simulink model "control_strategy_2"  (R2024b)
settings: Solver=VariableStepAuto  StartTime=0.0  StopTime=5  MaxStep=1e-3  MinStep=1e-9  RelTol=1e-3
values from neighbouring files (symbols this model uses):
  C_filtre = 1 / (Lc * (2 * pi * 2000)^2)    (= 2.53302959106e-06)    [acdc_converter_parameters.m]
  Ccb = 330e-6    (= 0.00033)    [dcdc_converter_parameters.m]
  Cdc = 2200e-6    (= 0.0022)    [acdc_converter_parameters.m]
  Ci = 220e-6    (= 0.00022)    [dcdc_converter_parameters.m]
  Is = P / Vac    [acdc_converter_parameters.m]
  KI_curr_d = 2 * pi * w_i * rac    [acdc_converter_main.m]
  KI_curr_q = 2 * pi * w_i * rac    [acdc_converter_main.m]
  KI_out = KP_out * Wci_out    [dcdc_converter_main.m]
  KI_volt = C_volt.Ki    [acdc_converter_main.m]
  KIi = KPi * Wci_out    [dcdc_converter_main.m]
  KP_curr_d = 2 * pi * w_i * Lc    [acdc_converter_main.m]
  KP_curr_q = 2 * pi * w_i * Lc    [acdc_converter_main.m]
  KP_out = Wbi_volt / (Giod * Wci_out)    [dcdc_converter_main.m]
  KP_q = C_q.Kp    [acdc_converter_main.m]
  KP_volt = C_volt.Kp    [acdc_converter_main.m]
  KPi = Wbi_dc / (DCGain_iod * Wci_out)    [dcdc_converter_main.m]
  Lb = 3e-3    (= 0.003)    [dcdc_converter_parameters.m]
  Lc = 2.5e-3    (= 0.0025)    [acdc_converter_parameters.m]
  Lsi = 105e-6    (= 0.000105)    [dcdc_converter_parameters.m]
  P = 500    [main_control_strategy_2.m]
  phase = 0    [acdc_converter_parameters.m]
  Q = 0    [main_control_strategy_2.m]
  rac = 1e-3    (= 0.001)    [acdc_converter_parameters.m]
  rb = 1e-3    (= 0.001)    [dcdc_converter_parameters.m]
  ro = 270e-3    (= 0.27)    [dcdc_converter_parameters.m]
  Vb = 48    [dcdc_converter_parameters.m]
  Vdc = 200    [acdc_converter_parameters.m]
  Vdc0 = Vdc    (= 200)    [acdc_converter_parameters.m]
  Vs0 = Vac    (= 120)    [acdc_converter_parameters.m]
  w = 2 * pi * f    (= 376.991118431)    [acdc_converter_parameters.m]
  Zl = w * Lc    (= 0.942477796077)    [acdc_converter_parameters.m]
undefined symbols (not defined in the file or in its folder): q_switch, ri
libraries: spsSeriesRLCBranchLib x8, slpidlib x6, spsMosfetLib x6, spsVoltageMeasurementLib x5, spsMeanLib x4, spsParallelRLCBranchLib x3, spsCurrentMeasurementLib x3, spsTHDLib x3, spsDCVoltageSourceLib x2, spsACVoltageSourceLib x1, spsGroundLib x1, spsPWMGenerator2LevelLib x1
settings Model: Creator=casti  LastModifiedBy=Asus
settings OptimizationCC: ReuseModelBlockBuffer=off
settings RTWCC: GPUComputeCapability=3.5

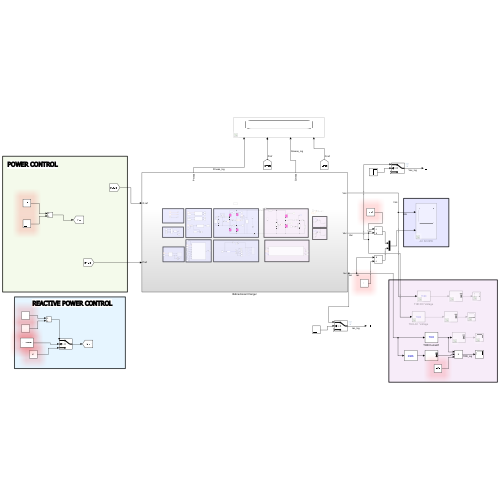
[thumbnail: Simulink's stored preview of the top-level diagram]
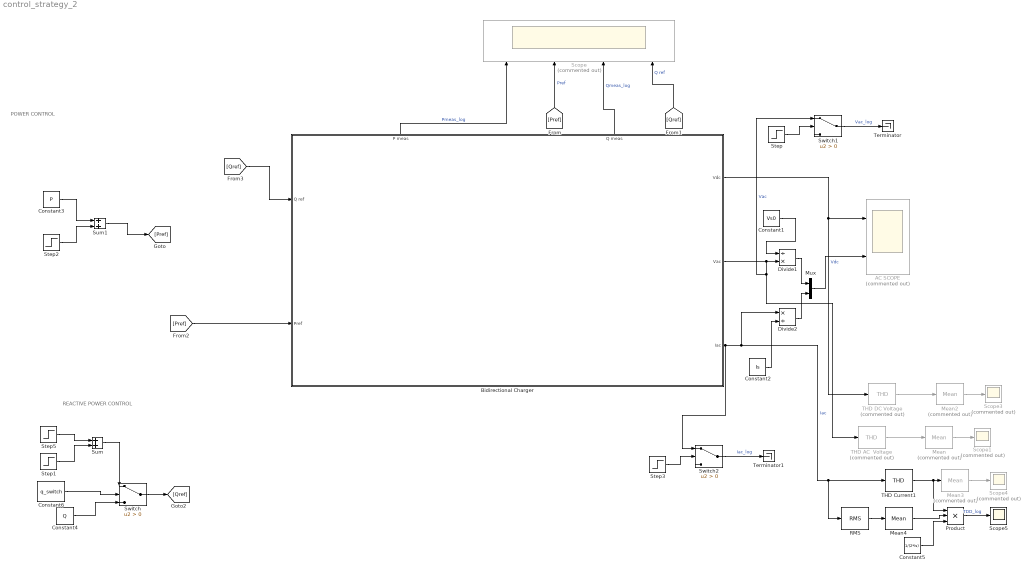
== system control_strategy_2 ==
  note: POWER CONTROL
  note: REACTIVE POWER CONTROL
  AC SCOPE : Scope  Commented=on  NumInputPorts=2
  Bidirectional Charger : Subsystem
      settings: PortSchema="{\"entries\":[{\"content\":{\"sides\":[{\"content\":{\"connectorIds\":[\"In1\",\"In2\"]},\"type\":\"ConnectorPlacement.EquallySpacedRectSide\",\"uuid\":\"0e8ef780-485e-4c8b-9a8b-f034f795c892\"},{\"content\":{\"connectorIds\":[\"Out1\",\"Out2\",\"Out3\"],\"side\":\"RIGHT\"},\"type\":\"ConnectorPlacement.EquallySpacedRectSide\",\"uuid\":\"9fd702af-2122-4ac4-9fd2-64e19671b5dd\"},{\"content\":{\"connectorIds\":[\"Out4\",\"Out5\"],\"side\":\"TOP\"},\"type\":\"ConnectorPlacement.EquallySpacedRectSide\",\"uuid\":\"331bdb16-1cb1-49e4-96bf-e66e7b38baa0\"}]},\"type\":\"ConnectorPlacement.EquallySpacedConnector\",\"uuid\":\"78325ce0-b63a-4b2a-b520-d47ca5f2449f\"}],\"packageUris\":[\"http://schema.mathworks.com/mf0/Connector/R2020b\"],\"version\":\"1.0\"}"
  Constant1 : Constant  Value=Vs0
  Constant2 : Constant  Value=Is
  Constant3 : Constant  Value=P
  Constant4 : Constant  Value=Q
  Constant5 : Constant  Value=1/(2*Is)
  Constant6 : Constant  Value=q_switch
  Divide1 : Product  Inputs=/*
  Divide2 : Product  Inputs=*/
  Mean : spsMeanLib/Mean  Commented=on  Freq=60  Vinit=0  Ts=0
  Mean2 : spsMeanLib/Mean  Commented=on  Freq=120  Vinit=0  Ts=0
  Mean3 : spsMeanLib/Mean  Commented=on  Freq=60  Vinit=0  Ts=0
  Mean4 : spsMeanLib/Mean  Freq=60  Vinit=0  Ts=0
  Mux : Mux  Inputs=2
  Product : Product  Inputs=3
  RMS : spsRMSLib/RMS  TrueRMS=on  Freq=60  RMSInit=120  Ts=0
  Scope : Scope  Commented=on  NumInputPorts=4
  Scope1 : Scope  Commented=on
  Scope3 : Scope  Commented=on
  Scope4 : Scope  Commented=on
  Scope5 : Scope
  Step : Step  Time=4.5  SampleTime=0
  Step1 : Step  Time=10  After=-2*Q  SampleTime=0
  Step2 : Step  Time=10  After=-2*P  SampleTime=0
  Step3 : Step  Time=4.5  SampleTime=0
  Step5 : Step  Time=0.05  After=Q  SampleTime=0
  Sum : Sum
  Sum1 : Sum
  Switch : Switch  Criteria=u2 > Threshold  SaturateOnIntegerOverflow=off  InputSameDT=off
  Switch1 : Switch  Criteria=u2 > Threshold  SaturateOnIntegerOverflow=off  InputSameDT=off
  Switch2 : Switch  Criteria=u2 > Threshold  SaturateOnIntegerOverflow=off  InputSameDT=off
  THD AC  Voltage : spsTHDLib/THD  Commented=on  Freq=60  Ts=0
  THD Current1 : spsTHDLib/THD  Freq=60  Ts=0
  THD DC Voltage : spsTHDLib/THD  Commented=on  Freq=120  Ts=0
  Terminator : Terminator
  Terminator1 : Terminator
  wires:
  Bidirectional Charger/4(P meas) -> Scope/1  "Pmeas_log"
  Bidirectional Charger/5(Q meas) -> Scope/3  "Qmeas_log"
  Mux/1 -> AC SCOPE/2
  Constant1/1 -> Divide1/1
  Constant2/1 -> Divide2/2
  Divide2/1 -> Mux/2
  Divide1/1 -> Mux/1
  [Qref] -> Scope/4  "Q ref"
  [Pref] -> Scope/2  "Pref"
  Mean/1 -> Scope1/1
  THD DC Voltage/1 -> Mean2/1
  Bidirectional Charger/1(Vdc) -> THD DC Voltage/1, AC SCOPE/1  "Vdc"
  THD AC  Voltage/1 -> Mean/1
  Bidirectional Charger/3(Iac) -> Switch2/1, RMS/1, THD Current1/1, Divide2/1  "Iac"
  Mean2/1 -> Scope3/1
  Bidirectional Charger/2(Vac) -> THD AC  Voltage/1, Switch1/1, Divide1/2  "Vac"
  [Pref] -> Bidirectional Charger/2(Pref)
  [Qref] -> Bidirectional Charger/1(Q ref)
  RMS/1 -> Mean4/1
  Constant5/1 -> Product/3
  THD Current1/1 -> Product/1, Mean3/1
  Mean3/1 -> Scope4/1
  Product/1 -> Scope5/1  "TDD_log"
  Mean4/1 -> Product/2
  Constant4/1 -> Switch/3
  Switch/1 -> [Qref]
  Constant6/1 -> Switch/2
  Sum/1 -> Switch/1
  Constant3/1 -> Sum1/1
  Step2/1 -> Sum1/2
  Sum1/1 -> [Pref]
  Step1/1 -> Sum/2
  Step5/1 -> Sum/1
  Step/1 -> Switch1/2
  Switch1/1 -> Terminator/1  "Vac_log"
  Step3/1 -> Switch2/2
  Switch2/1 -> Terminator1/1  "Iac_log"

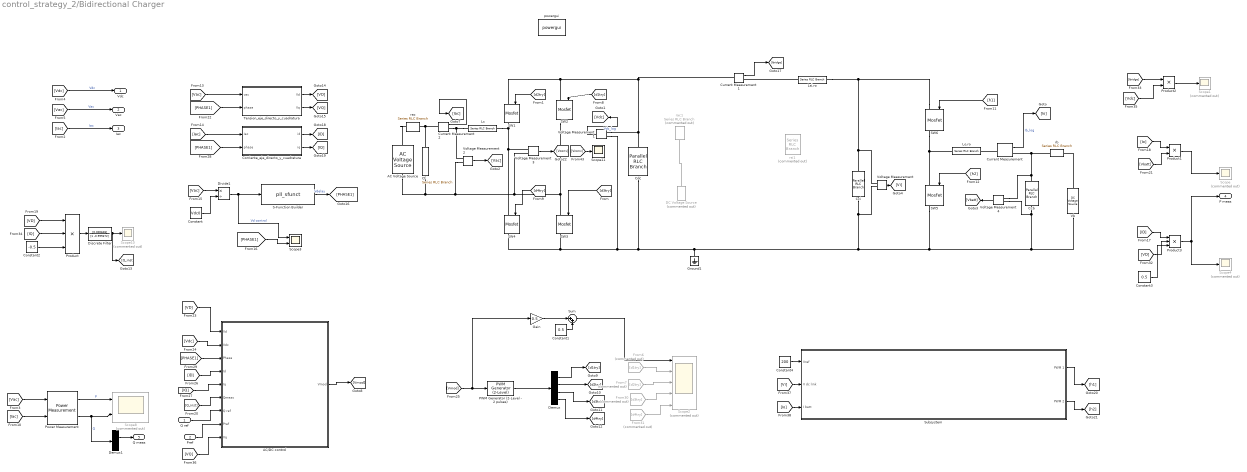
== system control_strategy_2/Bidirectional Charger ==
  Q ref : Inport
  Pref : Inport  Port=2
  AC Voltage Source : spsACVoltageSourceLib/AC Voltage Source  Amplitude=Vs0*sqrt(2)  Phase=0  Frequency=60  SampleTime=0  Measurements=None  BusType=swing  Pref=10e3  Qref=0  Qmin=-inf  Qmax=+inf
  AC/DC control : Subsystem
  Ccb : spsParallelRLCBranchLib/Parallel RLC Branch  LConnTagsString=a  RConnTagsString=__new0  BranchType=C  Resistance=1  Inductance=1e-3  SetiL0=off  InitialCurrent=0  Capacitance=Ccb  Setx0=on  InitialVoltage=Vb  Measurements=None
  Cci : spsParallelRLCBranchLib/Parallel RLC Branch  LConnTagsString=a  RConnTagsString=__new0  BranchType=C  Resistance=1  Inductance=1e-3  SetiL0=off  InitialCurrent=0  Capacitance=Ci  Setx0=on  InitialVoltage=Vsi  Measurements=None
  Cdc : spsParallelRLCBranchLib/Parallel RLC Branch  LConnTagsString=a  RConnTagsString=__new0  BranchType=C  Resistance=1  Inductance=1e-3  SetiL0=off  InitialCurrent=0  Capacitance=Cdc  Setx0=on  InitialVoltage=Vsi  Measurements=None
  Cf : spsSeriesRLCBranchLib/Series RLC Branch  LConnTagsString=__new0  RConnTagsString=__new0  BranchType=C  Resistance=rac  Inductance=Lc  SetiL0=off  InitialCurrent=Io0  Capacitance=C_filtre  Setx0=off  InitialVoltage=0  Measurements=None
  Constant : Constant  Value=Vdc0
  Constant1 : Constant  Value=0.5
  Constant2 : Constant  Value=-0.5
  Constant3 : Constant  Value=0.5
  Constant4 : Constant  Value=200
  Corriente_eje_directo_y_cuadratura : Subsystem
  Current Measurement : spsCurrentMeasurementLib/Current Measurement  PhasorSimulation=off  OutputType=Complex  PSBequivalent=0
  Current Measurement1 : spsCurrentMeasurementLib/Current Measurement  PhasorSimulation=off  OutputType=Complex  PSBequivalent=0
  Current Measurement2 : spsCurrentMeasurementLib/Current Measurement  PhasorSimulation=off  OutputType=Complex  PSBequivalent=0
  DC Voltage Source : spsDCVoltageSourceLib/DC Voltage Source  Commented=on  Amplitude=Vdc  Measurements=None
  Demux : Demux
  Demux1 : Demux
  Discrete Filter : DiscreteFilter  Numerator=[0.000628]  Denominator=[1 -0.999372]
  Divide1 : Product  Inputs=*/
  From30 : From  Commented=on  GotoTag=d3try
  From31 : From  Commented=on  GotoTag=d4try
  From6 : From  Commented=on  GotoTag=d1try
  From7 : From  Commented=on  GotoTag=d2try
  Gain : Gain  Gain=0.5
  Ground1 : spsGroundLib/Ground  LConnTagsString=a
  Lc : spsSeriesRLCBranchLib/Series RLC Branch  LConnTagsString=__new0  RConnTagsString=__new0  BranchType=L  Resistance=rac  Inductance=Lc  SetiL0=off  InitialCurrent=Io0  Capacitance=1e-6  Setx0=off  InitialVoltage=0  Measurements=None
  Lo,ro : spsSeriesRLCBranchLib/Series RLC Branch  LConnTagsString=__new0  RConnTagsString=__new0  BranchType=RL  Resistance=ro  Inductance=Lb  SetiL0=off  InitialCurrent=Io0  Capacitance=1e-6  Setx0=off  InitialVoltage=0  Measurements=None
  Lsi,ro : spsSeriesRLCBranchLib/Series RLC Branch  LConnTagsString=__new0  RConnTagsString=__new0  BranchType=RL  Resistance=ro  Inductance=Lsi  SetiL0=off  InitialCurrent=Io0  Capacitance=1e-6  Setx0=off  InitialVoltage=0  Measurements=None
  PWM Generator (2-Level - 2 pulses) : spsPWMGenerator2LevelLib/PWM Generator (2-Level)  ModulatorType=Single-phase full-bridge - Bipolar modulation (4 pulses)  ModulatorMode=Unsynchronized  Fc=20000  Pc=90  nF=27  MinMax="[ -1  1 ]"  SamplingTechnique=Natural  ModulatingSignals=off  m=0.6  Freq=60  Phase=30  Ts=5e-7  ShowCarrierOutport=off
  Power Measurement : eePowerMeasurement/Power Measurement  LabelModeActiveChoice=Continuous  F=60  K=[0 1 2 3]  Ts=0
  Product : Product  Inputs=3
  Product1 : Product
  Product2 : Product
  Product3 : Product  Inputs=3
  S-Function Builder : S-Function  FunctionName=pll_sfunct  SFunctionModules=pll_sfunct_wrapper.c  SFunctionDeploymentMode=off  EnableBusSupport=off  mask(S-Function Builder){}
      mask help: Simulink:masks:SFunctionBuilder_MD
      mask init:
      | val = [[.9  0.75 0.75 1 1 .9 .9 1]',[1 1 0.75 0.75 .9 .9 1 .9]'];try , sys = get_param(gcb,'SfunBuilderFcnName');if isempty(sys), sys = get_param(gcb,'FunctionName'); end,catch, sys = get_param(gcb,'FunctionName'); end
      settings: CopyFcn=set_param(gcbh,'LinkStatus','none')  OpenFcn=sfunctionwizard(gcbh)
      mask Display:
      | plot(val(:,1),val(:,2))
      | disp(sys)
      | port_label('input',1,sprintf('%s', 'Vac'),'interpreter','tex')
      | port_label('output',1,sprintf('%s', 'phase'),'interpreter','tex')
  SW{1..6} (6 alike) : spsMosfetLib/Mosfet  Ron=1e-3  Lon=0  Rd=0.00001  Vfd=0  IC=0  Rs=1e5  Cs=inf  Measurements=on
  Scope{,1,4,10} (4 alike) : Scope  Commented=on
  Scope11 : Scope
  Scope2 : Scope  Commented=on  NumInputPorts=5
  Scope3 : Scope  NumInputPorts=2
  Scope8 : Scope  Commented=on  NumInputPorts=2
  Subsystem : Subsystem
  Sum : Sum  Inputs=|++
  Tension_eje_directo_y_cuadratura : Subsystem
  Vb : spsDCVoltageSourceLib/DC Voltage Source  Amplitude=Vb  Measurements=None
  Voltage Measurement{,1..4} (5 alike) : spsVoltageMeasurementLib/Voltage Measurement  PhasorSimulation=off  OutputType=Complex  PSBequivalent=0
  powergui : spspowerguiLib/powergui  Priority=1  SimulationMode=Discrete  SampleTime=5e-7  frequency=60  Iterations=50  frequencyindice=0  Pbase=100e6  ErrMax=1e-4  UnitsV=kV  UnitsW=MW  buscounter=0  FunctionMessages=off  echomessages=off  EnableUseOfTLC=off  CurrentSourceSwitches=off  DisableSnubberDevices=off  DisableRonSwitches=off  DisableVfSwitches=off  DisplayEquations=off  AutomaticDiscreteSolvers=off  SolverType=Tustin/Backward Euler (TBE)  Interpol=off  ExternalGateDelay=off  methode=off  Ts=100  x0status=blocks  SPID=on  SwTol=0  HookPort=off  NonlinearTolerance=1e-4  nMaxIteration=100  ContinueOnMaxIteration=off  RestoreLinks=warning  ResistiveCurrentMeasurement=off  Frange=[0:2:500]  Ylog=off  Xlog=on  ShowGrid=off  save=off  variable=ZData  structure=0  ZoomFFT=off  StartTime=0.0  cycles=1  DisplayStyle=1  fundamental=60  FreqAxis=off  MaxFrequency=1000  frequencyindicesteady=1  RmsSteady=1  display=off
  rac : spsSeriesRLCBranchLib/Series RLC Branch  LConnTagsString=__new0  RConnTagsString=__new0  BranchType=R  Resistance=rac  Inductance=Lc  SetiL0=off  InitialCurrent=Io0  Capacitance=1e-6  Setx0=off  InitialVoltage=0  Measurements=None
  rac1 : spsSeriesRLCBranchLib/Series RLC Branch  Commented=on  LConnTagsString=__new0  RConnTagsString=__new0  BranchType=R  Resistance=rac  Inductance=Lc  SetiL0=off  InitialCurrent=Io0  Capacitance=1e-6  Setx0=off  InitialVoltage=0  Measurements=None
  rb : spsSeriesRLCBranchLib/Series RLC Branch  LConnTagsString=__new0  RConnTagsString=__new0  BranchType=R  Resistance=rb  Inductance=1e-3  SetiL0=off  InitialCurrent=0  Capacitance=1e-6  Setx0=off  InitialVoltage=0  Measurements=None
  rsi1 : spsSeriesRLCBranchLib/Series RLC Branch  Commented=on  LConnTagsString=__new0  RConnTagsString=__new0  BranchType=R  Resistance=ri  Inductance=1e-3  SetiL0=off  InitialCurrent=0  Capacitance=1e-6  Setx0=off  InitialVoltage=0  Measurements=None
  Vdc : Outport
  Vac : Outport  Port=2
  Iac : Outport  Port=3
  P meas : Outport  Port=4
  Q meas : Outport  Port=5
  wires:
  From7/1 -> Scope2/3
  Voltage Measurement3/1 -> [Vconv]
  PWM Generator (2-Level - 2 pulses)/1 -> Demux/1
  [Vconv] -> Scope11/1
  [PHASE1] -> Corriente_eje_directo_y_cuadratura/2(phase)
  [h1] -> SW6/1
  [Vac] -> Vac/1  "Vac"
  [Vac] -> Divide1/1
  AC/DC control/1(Vmod) -> [Vmod]
  Tension_eje_directo_y_cuadratura/1(Vd) -> [VD]
  Gain/1 -> Sum/1
  [Iac] -> Corriente_eje_directo_y_cuadratura/1(Iac)
  Divide1/1 -> Scope3/1, S-Function Builder/1  "Vd control"
  Sum/1 -> Scope2/1
  Current Measurement2/1 -> [Iac]
  Voltage Measurement/1 -> [Vi]
  Voltage Measurement1/1 -> [Vdc]  "Vdc_log"
  Current Measurement/1 -> [Io]  "Ib_log"
  [d2try] -> SW1/1
  Demux/4 -> [d4try]
  Constant1/1 -> Sum/2
  [Vdc] -> Vdc/1  "Vdc"
  [d1try] -> SW2/1
  Constant/1 -> Divide1/2
  From31/1 -> Scope2/5
  [d3try] -> SW3/1
  S-Function Builder/1 -> [PHASE1]  "Vdelay"
  Voltage Measurement2/1 -> [Vac]
  Demux/1 -> [d1try]
  [Vmod] -> Gain/1, PWM Generator (2-Level - 2 pulses)/1
  [d4try] -> SW4/1
  [Vac] -> Tension_eje_directo_y_cuadratura/1(vac)
  Tension_eje_directo_y_cuadratura/2(Vq) -> [VQ]
  Corriente_eje_directo_y_cuadratura/1(id) -> [ID]
  Corriente_eje_directo_y_cuadratura/2(iq) -> [IQ]
  [PHASE1] -> Scope3/2
  [PHASE1] -> Tension_eje_directo_y_cuadratura/2(phase)
  [Iac] -> Iac/1  "Iac"
  [ID] -> AC/DC control/4(Id)
  Demux/2 -> [d2try]
  Demux/3 -> [d3try]
  From30/1 -> Scope2/4
  From6/1 -> Scope2/2
  [Vdc] -> AC/DC control/2(Vdc)
  [VD] -> AC/DC control/1(Vd)
  [IQ] -> AC/DC control/5(Iq)
  [PHASE1] -> AC/DC control/3(Phase)
  Power Measurement/2 -> Demux1/1, Scope8/2  "Q"
  [Iac] -> Power Measurement/2
  Demux1/2 -> Q meas/1
  Power Measurement/1 -> Scope8/1  "P"
  [Vac] -> Power Measurement/1
  [Q_inst] -> AC/DC control/6(Qmeas)
  [VD] -> Product/1
  Discrete Filter/1 -> [Q_inst], Scope10/1
  Product/1 -> Discrete Filter/1
  [IQ] -> Product/2
  Constant2/1 -> Product/3
  Q ref/1 -> AC/DC control/7(Q ref)
  Voltage Measurement4/1 -> [Vbatt]
  [Io] -> Product1/1
  [Vbatt] -> Product1/2
  Product1/1 -> Scope/1
  [h2] -> SW5/1
  Pref/1 -> AC/DC control/8(Pref)
  Current Measurement1/1 -> [Ibridge]
  [Ibridge] -> Product2/1
  [Vdc] -> Product2/2
  Product2/1 -> Scope1/1
  [VQ] -> AC/DC control/9(Vq)
  Constant4/1 -> Subsystem/1(Vref)
  [Vi] -> Subsystem/2(V dc link)
  [Io] -> Subsystem/3(I batt)
  Subsystem/1(PWM 1) -> [h1]
  Subsystem/2(PWM 2) -> [h2]
  Product3/1 -> P meas/1, Scope4/1
  [VD] -> Product3/2
  [ID] -> Product3/1
  Constant3/1 -> Product3/3
  connections:
  SW4/LConn1 -- Lc/RConn1 -- SW1/RConn1 -- Voltage Measurement3/LConn1
  SW6/LConn1 -- Cci/LConn1 -- Voltage Measurement/LConn1 -- Lsi,ro/LConn1
  SW2/LConn1 -- Current Measurement1/LConn1 -- Cdc/LConn1 -- Voltage Measurement1/LConn1 -- SW1/LConn1
  Voltage Measurement4/LConn2 -- Cci/RConn1 -- Voltage Measurement/LConn2 -- Voltage Measurement1/LConn2 -- SW4/RConn1 -- SW3/RConn1 -- Cdc/RConn1 -- Ground1/LConn1 -- SW5/RConn1 -- Vb/LConn1 -- Ccb/RConn1
  Vb/RConn1 -- rb/RConn1
  SW6/RConn1 -- SW5/LConn1 -- Lo,ro/LConn1
  rac/LConn1 -- Current Measurement2/LConn1 -- Cf/LConn1
  Voltage Measurement2/LConn2 -- AC Voltage Source/LConn1 -- Cf/RConn1 -- SW2/RConn1 -- SW3/LConn1 -- Voltage Measurement3/LConn2
  Ccb/LConn1 -- rb/LConn1 -- Current Measurement/RConn1 -- Voltage Measurement4/LConn1
  Current Measurement/LConn1 -- Lo,ro/RConn1
  Lc/LConn1 -- Current Measurement2/RConn1 -- Voltage Measurement2/LConn1
  rac/RConn1 -- AC Voltage Source/RConn1
  DC Voltage Source/RConn1 -- rac1/LConn1
  Lsi,ro/RConn1 -- Current Measurement1/RConn1

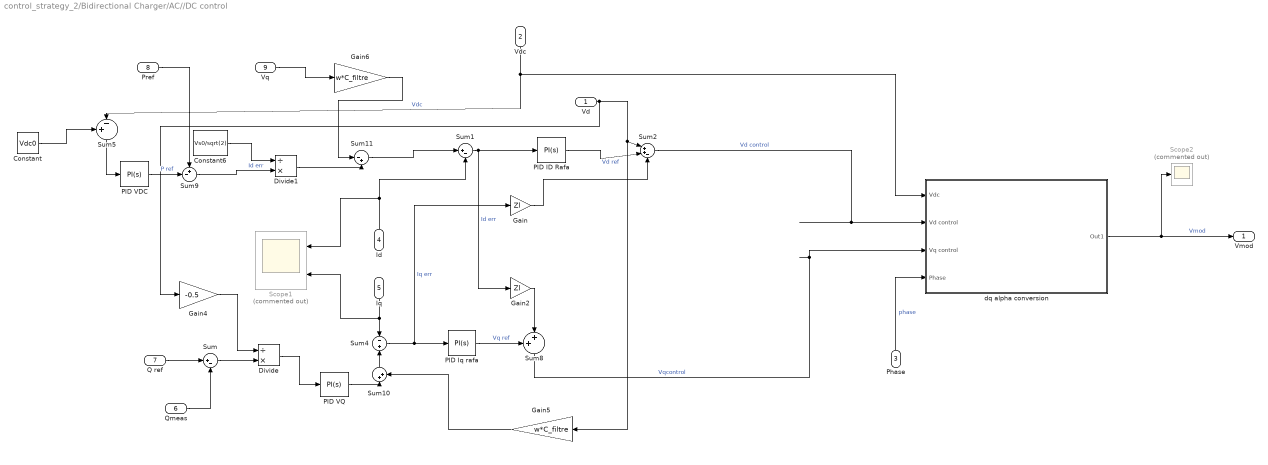
== system control_strategy_2/Bidirectional Charger/AC//DC control ==
  Vd : Inport
  Vdc : Inport  Port=2
  Phase : Inport  Port=3
  Id : Inport  Port=4
  Iq : Inport  Port=5
  Qmeas : Inport  Port=6
  Q ref : Inport  Port=7
  Pref : Inport  Port=8
  Vq : Inport  Port=9
  Constant : Constant  Value=Vdc0
  Constant6 : Constant  Value=Vs0/sqrt(2)
  Divide : Product  Inputs=/*
  Divide1 : Product  Inputs=/*
  Gain : Gain  Gain=Zl
  Gain2 : Gain  Gain=Zl
  Gain4 : Gain  Gain=-0.5
  Gain5 : Gain  Gain=w*C_filtre
  Gain6 : Gain  Gain=w*C_filtre
  PID ID Rafa : slpidlib/PID Controller  Controller=PI  Form=Parallel  TimeDomain=Continuous-time  UseExternalTs=off  SampleTime=-1  IntegratorMethod=Forward Euler  FilterMethod=Forward Euler  ControllerParametersSource=internal  P=KP_curr_d  I=KI_curr_d  UseKiTs=off  D=0  UseExternalDerivativeSource=off  N=100  UseFilter=on  TunerSelectOption=Transfer Function Based (PID Tuner App)  InitialConditionSource=internal  InitialConditionForIntegrator=0  InitialConditionForFilter=0  DifferentiatorICPrevScaledInput=0  ExternalReset=none  TrackingMode=off  Kt=1  LimitOutput=off  SatLimitsSource=internal  UpperSaturationLimit=300  LowerSaturationLimit=0  LinearizeAsGain=on  AntiWindupMode=none  Kb=1  LimitIntegrator=off  UpperIntegratorSaturationLimit=inf  LowerIntegratorSaturationLimit=-inf  POutMin=[]  POutMax=[]  IOutMin=[]  IOutMax=[]  DOutMin=[]  DOutMax=[]  NOutMin=[]  NOutMax=[]  SumOutMin=[]  SumOutMax=[]  SaturationOutMin=[]  SaturationOutMax=[]  PParamMin=[]  PParamMax=[]  IParamMin=[]  IParamMax=[]  DParamMin=[]  DParamMax=[]  NParamMin=[]  NParamMax=[]  KbParamMin=[]  KbParamMax=[]  KtParamMin=[]  KtParamMax=[]  KbOutMin=[]  KbOutMax=[]  KtOutMin=[]  KtOutMax=[]  IntegratorOutMin=[]  IntegratorOutMax=[]  FilterOutMin=[]  FilterOutMax=[]  SumI1OutMin=[]  SumI1OutMax=[]  SumI2OutMin=[]  SumI2OutMax=[]  SumI3OutMin=[]  SumI3OutMax=[]  SumI4OutMin=[]  SumI4OutMax=[]  SumDOutMin=[]  SumDOutMax=[]  DifferentiatorOutMin=[]  DifferentiatorOutMax=[]  FilterDiffOutCoefMin=[]  FilterDiffOutCoefMax=[]  ReciprocalOutMin=[]  ReciprocalOutMax=[]  SumDenOutMin=[]  SumDenOutMax=[]  SumNumOutMin=[]  SumNumOutMax=[]  DivideOutMin=[]  DivideOutMax=[]  UdiffTsProdOutMin=[]  UdiffTsProdOutMax=[]  NTsProdOutMin=[]  NTsProdOutMax=[]  UintegralTsProdOutMin=[]  UintegralTsProdOutMax=[]  UngainTsProdOutMin=[]  UngainTsProdOutMax=[]  ClampingZeroOutDataTypeStr=Inherit: Inherit via back propagation  ClampingZeroOutMin=[]  ClampingZeroOutMax=[]  FilterDenConstantOutDataTypeStr=Inherit: Inherit via back propagation  FilterDenConstantOutMin=[]  FilterDenConstantOutMax=[]  PCopyOutDataTypeStr=Inherit: Inherit via back propagation  PCopyOutMin=[]  PCopyOutMax=[]  NCopyOutDataTypeStr=Inherit: Inherit via back propagation  NCopyOutMin=[]  NCopyOutMax=[]  IntegratorContinuousStateAttributes=''  IntegratorStateMustResolveToSignalObject=off  IntegratorRTWStateStorageClass=Auto  FilterContinuousStateAttributes=''  FilterStateMustResolveToSignalObject=off  FilterRTWStateStorageClass=Auto  ParallelPVariant=InternalParameters  IdealPVariant=Disabled  IVariant=InternalParameters  DVariant=Disabled  IntegratorVariant=Continuous  SatVariant=Disabled  AWVariant=Passthrough  PCopyVariant=Disabled  TRVariant=Disabled  FdbkBlocksVariant=Forward  IdealPFdbkVariant=Disabled  SatFdbkVariant=Disabled  DerivativeFilterVariant=Disabled  NVariant=Disabled  NCopyVariant=Disabled_SignalSpec  FilterICVariant=Disabled  IntegratorICVariant=InternalICs  ExternalResetVariant=Disabled  TRSumVariant=Passthrough  SumFdbkVariant=Disabled  SumVariant=Sum_PI  TsampFilterVariant=InternalTs  TsampNgainVariant=Passthrough  TsampIntegralVariant=Disabled_SignalSpec  ExternalSaturationOutDataTypeStr=Inherit: Same as second input  DerivativeSourceVariant=Disabled  PreIntVariant=InternalPreInt
  PID Iq rafa : slpidlib/PID Controller  Controller=PI  Form=Parallel  TimeDomain=Continuous-time  UseExternalTs=off  SampleTime=-1  IntegratorMethod=Forward Euler  FilterMethod=Forward Euler  ControllerParametersSource=internal  P=KP_curr_q  I=KI_curr_q  UseKiTs=off  D=0  UseExternalDerivativeSource=off  N=100  UseFilter=on  TunerSelectOption=Transfer Function Based (PID Tuner App)  InitialConditionSource=internal  InitialConditionForIntegrator=0  InitialConditionForFilter=0  DifferentiatorICPrevScaledInput=0  ExternalReset=none  TrackingMode=off  Kt=1  LimitOutput=off  SatLimitsSource=internal  UpperSaturationLimit=50  LowerSaturationLimit=-50  LinearizeAsGain=on  AntiWindupMode=none  Kb=1  LimitIntegrator=off  UpperIntegratorSaturationLimit=inf  LowerIntegratorSaturationLimit=-inf  POutMin=[]  POutMax=[]  IOutMin=[]  IOutMax=[]  DOutMin=[]  DOutMax=[]  NOutMin=[]  NOutMax=[]  SumOutMin=[]  SumOutMax=[]  SaturationOutMin=[]  SaturationOutMax=[]  PParamMin=[]  PParamMax=[]  IParamMin=[]  IParamMax=[]  DParamMin=[]  DParamMax=[]  NParamMin=[]  NParamMax=[]  KbParamMin=[]  KbParamMax=[]  KtParamMin=[]  KtParamMax=[]  KbOutMin=[]  KbOutMax=[]  KtOutMin=[]  KtOutMax=[]  IntegratorOutMin=[]  IntegratorOutMax=[]  FilterOutMin=[]  FilterOutMax=[]  SumI1OutMin=[]  SumI1OutMax=[]  SumI2OutMin=[]  SumI2OutMax=[]  SumI3OutMin=[]  SumI3OutMax=[]  SumI4OutMin=[]  SumI4OutMax=[]  SumDOutMin=[]  SumDOutMax=[]  DifferentiatorOutMin=[]  DifferentiatorOutMax=[]  FilterDiffOutCoefMin=[]  FilterDiffOutCoefMax=[]  ReciprocalOutMin=[]  ReciprocalOutMax=[]  SumDenOutMin=[]  SumDenOutMax=[]  SumNumOutMin=[]  SumNumOutMax=[]  DivideOutMin=[]  DivideOutMax=[]  UdiffTsProdOutMin=[]  UdiffTsProdOutMax=[]  NTsProdOutMin=[]  NTsProdOutMax=[]  UintegralTsProdOutMin=[]  UintegralTsProdOutMax=[]  UngainTsProdOutMin=[]  UngainTsProdOutMax=[]  ClampingZeroOutDataTypeStr=Inherit: Inherit via back propagation  ClampingZeroOutMin=[]  ClampingZeroOutMax=[]  FilterDenConstantOutDataTypeStr=Inherit: Inherit via back propagation  FilterDenConstantOutMin=[]  FilterDenConstantOutMax=[]  PCopyOutDataTypeStr=Inherit: Inherit via back propagation  PCopyOutMin=[]  PCopyOutMax=[]  NCopyOutDataTypeStr=Inherit: Inherit via back propagation  NCopyOutMin=[]  NCopyOutMax=[]  IntegratorContinuousStateAttributes=''  IntegratorStateMustResolveToSignalObject=off  IntegratorRTWStateStorageClass=Auto  FilterContinuousStateAttributes=''  FilterStateMustResolveToSignalObject=off  FilterRTWStateStorageClass=Auto  ParallelPVariant=InternalParameters  IdealPVariant=Disabled  IVariant=InternalParameters  DVariant=Disabled  IntegratorVariant=Continuous  SatVariant=Disabled  AWVariant=Passthrough  PCopyVariant=Disabled  TRVariant=Disabled  FdbkBlocksVariant=Forward  IdealPFdbkVariant=Disabled  SatFdbkVariant=Disabled  DerivativeFilterVariant=Disabled  NVariant=Disabled  NCopyVariant=Disabled_SignalSpec  FilterICVariant=Disabled  IntegratorICVariant=InternalICs  ExternalResetVariant=Disabled  TRSumVariant=Passthrough  SumFdbkVariant=Disabled  SumVariant=Sum_PI  TsampFilterVariant=InternalTs  TsampNgainVariant=Passthrough  TsampIntegralVariant=Disabled_SignalSpec  ExternalSaturationOutDataTypeStr=Inherit: Same as second input  DerivativeSourceVariant=Disabled  PreIntVariant=InternalPreInt
  "PID VDC " : slpidlib/PID Controller  Controller=PI  Form=Parallel  TimeDomain=Continuous-time  UseExternalTs=off  SampleTime=-1  IntegratorMethod=Forward Euler  FilterMethod=Forward Euler  ControllerParametersSource=internal  P=KP_volt*0.10  I=KI_volt*0.10  UseKiTs=off  D=0  UseExternalDerivativeSource=off  N=100  UseFilter=on  TunerSelectOption=Frequency Response Based  InitialConditionSource=internal  InitialConditionForIntegrator=0  InitialConditionForFilter=0  DifferentiatorICPrevScaledInput=0  ExternalReset=none  TrackingMode=off  Kt=1  LimitOutput=on  SatLimitsSource=internal  UpperSaturationLimit=700  LowerSaturationLimit=-700  LinearizeAsGain=on  AntiWindupMode=none  Kb=1  LimitIntegrator=off  UpperIntegratorSaturationLimit=inf  LowerIntegratorSaturationLimit=-inf  POutMin=[]  POutMax=[]  IOutMin=[]  IOutMax=[]  DOutMin=[]  DOutMax=[]  NOutMin=[]  NOutMax=[]  SumOutMin=[]  SumOutMax=[]  SaturationOutMin=[]  SaturationOutMax=[]  PParamMin=[]  PParamMax=[]  IParamMin=[]  IParamMax=[]  DParamMin=[]  DParamMax=[]  NParamMin=[]  NParamMax=[]  KbParamMin=[]  KbParamMax=[]  KtParamMin=[]  KtParamMax=[]  KbOutMin=[]  KbOutMax=[]  KtOutMin=[]  KtOutMax=[]  IntegratorOutMin=[]  IntegratorOutMax=[]  FilterOutMin=[]  FilterOutMax=[]  SumI1OutMin=[]  SumI1OutMax=[]  SumI2OutMin=[]  SumI2OutMax=[]  SumI3OutMin=[]  SumI3OutMax=[]  SumI4OutMin=[]  SumI4OutMax=[]  SumDOutMin=[]  SumDOutMax=[]  DifferentiatorOutMin=[]  DifferentiatorOutMax=[]  FilterDiffOutCoefMin=[]  FilterDiffOutCoefMax=[]  ReciprocalOutMin=[]  ReciprocalOutMax=[]  SumDenOutMin=[]  SumDenOutMax=[]  SumNumOutMin=[]  SumNumOutMax=[]  DivideOutMin=[]  DivideOutMax=[]  UdiffTsProdOutMin=[]  UdiffTsProdOutMax=[]  NTsProdOutMin=[]  NTsProdOutMax=[]  UintegralTsProdOutMin=[]  UintegralTsProdOutMax=[]  UngainTsProdOutMin=[]  UngainTsProdOutMax=[]  ClampingZeroOutDataTypeStr=Inherit: Inherit via back propagation  ClampingZeroOutMin=[]  ClampingZeroOutMax=[]  FilterDenConstantOutDataTypeStr=Inherit: Inherit via back propagation  FilterDenConstantOutMin=[]  FilterDenConstantOutMax=[]  PCopyOutDataTypeStr=Inherit: Inherit via back propagation  PCopyOutMin=[]  PCopyOutMax=[]  NCopyOutDataTypeStr=Inherit: Inherit via back propagation  NCopyOutMin=[]  NCopyOutMax=[]  IntegratorContinuousStateAttributes=''  IntegratorStateMustResolveToSignalObject=off  IntegratorRTWStateStorageClass=Auto  FilterContinuousStateAttributes=''  FilterStateMustResolveToSignalObject=off  FilterRTWStateStorageClass=Auto  ParallelPVariant=InternalParameters  IdealPVariant=Disabled  IVariant=InternalParameters  DVariant=Disabled  IntegratorVariant=Continuous  SatVariant=Enabled  AWVariant=Passthrough  PCopyVariant=Disabled  TRVariant=Disabled  FdbkBlocksVariant=Forward  IdealPFdbkVariant=Disabled  SatFdbkVariant=Disabled  DerivativeFilterVariant=Disabled  NVariant=Disabled  NCopyVariant=Disabled_SignalSpec  FilterICVariant=Disabled  IntegratorICVariant=InternalICs  ExternalResetVariant=Disabled  TRSumVariant=Passthrough  SumFdbkVariant=Disabled  SumVariant=Sum_PI  TsampFilterVariant=InternalTs  TsampNgainVariant=Passthrough  TsampIntegralVariant=Disabled_SignalSpec  ExternalSaturationOutDataTypeStr=Inherit: Same as second input  DerivativeSourceVariant=Disabled  PreIntVariant=InternalPreInt
  PID VQ : slpidlib/PID Controller  Controller=PI  Form=Parallel  TimeDomain=Continuous-time  UseExternalTs=off  SampleTime=-1  IntegratorMethod=Forward Euler  FilterMethod=Forward Euler  ControllerParametersSource=internal  P=KP_q+0.08  I=50  UseKiTs=off  D=0  UseExternalDerivativeSource=off  N=100  UseFilter=on  TunerSelectOption=Frequency Response Based  InitialConditionSource=internal  InitialConditionForIntegrator=0  InitialConditionForFilter=0  DifferentiatorICPrevScaledInput=0  ExternalReset=none  TrackingMode=off  Kt=1  LimitOutput=off  SatLimitsSource=internal  UpperSaturationLimit=16  LowerSaturationLimit=-16  LinearizeAsGain=on  AntiWindupMode=none  Kb=1  LimitIntegrator=off  UpperIntegratorSaturationLimit=inf  LowerIntegratorSaturationLimit=-inf  POutMin=[]  POutMax=[]  IOutMin=[]  IOutMax=[]  DOutMin=[]  DOutMax=[]  NOutMin=[]  NOutMax=[]  SumOutMin=[]  SumOutMax=[]  SaturationOutMin=[]  SaturationOutMax=[]  PParamMin=[]  PParamMax=[]  IParamMin=[]  IParamMax=[]  DParamMin=[]  DParamMax=[]  NParamMin=[]  NParamMax=[]  KbParamMin=[]  KbParamMax=[]  KtParamMin=[]  KtParamMax=[]  KbOutMin=[]  KbOutMax=[]  KtOutMin=[]  KtOutMax=[]  IntegratorOutMin=[]  IntegratorOutMax=[]  FilterOutMin=[]  FilterOutMax=[]  SumI1OutMin=[]  SumI1OutMax=[]  SumI2OutMin=[]  SumI2OutMax=[]  SumI3OutMin=[]  SumI3OutMax=[]  SumI4OutMin=[]  SumI4OutMax=[]  SumDOutMin=[]  SumDOutMax=[]  DifferentiatorOutMin=[]  DifferentiatorOutMax=[]  FilterDiffOutCoefMin=[]  FilterDiffOutCoefMax=[]  ReciprocalOutMin=[]  ReciprocalOutMax=[]  SumDenOutMin=[]  SumDenOutMax=[]  SumNumOutMin=[]  SumNumOutMax=[]  DivideOutMin=[]  DivideOutMax=[]  UdiffTsProdOutMin=[]  UdiffTsProdOutMax=[]  NTsProdOutMin=[]  NTsProdOutMax=[]  UintegralTsProdOutMin=[]  UintegralTsProdOutMax=[]  UngainTsProdOutMin=[]  UngainTsProdOutMax=[]  ClampingZeroOutDataTypeStr=Inherit: Inherit via back propagation  ClampingZeroOutMin=[]  ClampingZeroOutMax=[]  FilterDenConstantOutDataTypeStr=Inherit: Inherit via back propagation  FilterDenConstantOutMin=[]  FilterDenConstantOutMax=[]  PCopyOutDataTypeStr=Inherit: Inherit via back propagation  PCopyOutMin=[]  PCopyOutMax=[]  NCopyOutDataTypeStr=Inherit: Inherit via back propagation  NCopyOutMin=[]  NCopyOutMax=[]  IntegratorContinuousStateAttributes=''  IntegratorStateMustResolveToSignalObject=off  IntegratorRTWStateStorageClass=Auto  FilterContinuousStateAttributes=''  FilterStateMustResolveToSignalObject=off  FilterRTWStateStorageClass=Auto  ParallelPVariant=InternalParameters  IdealPVariant=Disabled  IVariant=InternalParameters  DVariant=Disabled  IntegratorVariant=Continuous  SatVariant=Disabled  AWVariant=Passthrough  PCopyVariant=Disabled  TRVariant=Disabled  FdbkBlocksVariant=Forward  IdealPFdbkVariant=Disabled  SatFdbkVariant=Disabled  DerivativeFilterVariant=Disabled  NVariant=Disabled  NCopyVariant=Disabled_SignalSpec  FilterICVariant=Disabled  IntegratorICVariant=InternalICs  ExternalResetVariant=Disabled  TRSumVariant=Passthrough  SumFdbkVariant=Disabled  SumVariant=Sum_PI  TsampFilterVariant=InternalTs  TsampNgainVariant=Passthrough  TsampIntegralVariant=Disabled_SignalSpec  ExternalSaturationOutDataTypeStr=Inherit: Same as second input  DerivativeSourceVariant=Disabled  PreIntVariant=InternalPreInt
  Scope1 : Scope  Commented=on  NumInputPorts=2
  Scope2 : Scope  Commented=on
  Sum : Sum  Inputs=|+-
  Sum1 : Sum  Inputs=|+-
  Sum10 : Sum  Inputs=|++
  Sum11 : Sum  Inputs=|-+
  Sum2 : Sum  Inputs=|++-
  Sum4 : Sum  Inputs=-+
  Sum5 : Sum  Inputs=+-|
  Sum8 : Sum  Inputs=++|
  Sum9 : Sum  Inputs=+-|
  dq alpha conversion : Subsystem
  Vmod : Outport
  wires:
  Constant/1 -> Sum5/1
  Sum4/1 -> PID Iq rafa/1, Gain/1  "Iq err"
  Sum1/1 -> PID ID Rafa/1, Gain2/1  "Id err"
  PID Iq rafa/1 -> Sum8/1  "Vq ref"
  Phase/1 -> dq alpha conversion/4(Phase)  "phase"
  PID ID Rafa/1 -> Sum2/2  "Vd ref"
  Vdc/1 -> dq alpha conversion/1(Vdc), Sum5/2  "Vdc"
  dq alpha conversion/1(Out1) -> Scope2/1, Vmod/1  "Vmod"
  Gain/1 -> Sum2/3
  Gain2/1 -> Sum8/2
  Id/1 -> Scope1/1, Sum1/2
  Iq/1 -> Scope1/2, Sum4/1
  Sum2/1 -> dq alpha conversion/2(Vd control)  "Vd control"
  Sum8/1 -> dq alpha conversion/3(Vq control)  "Vqcontrol"
  Vd/1 -> Gain4/1, Gain5/1, Sum2/1
  Gain4/1 -> Divide/1
  Divide/1 -> PID VQ/1
  Sum/1 -> Divide/2
  Qmeas/1 -> Sum/2
  Q ref/1 -> Sum/1
  "PID VDC "/1 -> Sum9/2  "P ref"
  Constant6/1 -> Divide1/1
  Sum5/1 -> "PID VDC "/1
  Pref/1 -> Sum9/1
  Sum9/1 -> Divide1/2  "Id err"
  Sum10/1 -> Sum4/2
  PID VQ/1 -> Sum10/1
  Gain5/1 -> Sum10/2
  Vq/1 -> Gain6/1
  Divide1/1 -> Sum11/2
  Gain6/1 -> Sum11/1
  Sum11/1 -> Sum1/1

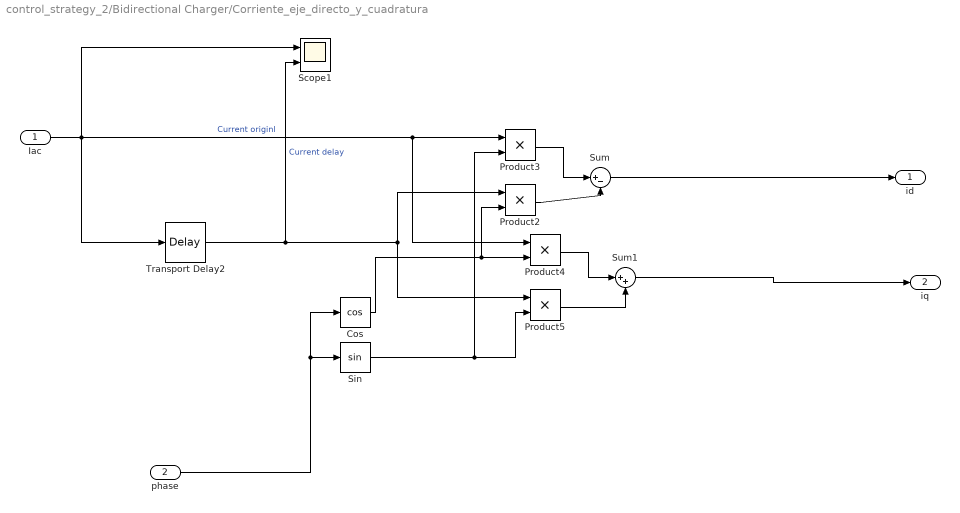
== system control_strategy_2/Bidirectional Charger/Corriente_eje_directo_y_cuadratura ==
  Iac : Inport
  phase : Inport  Port=2
  Cos : Trigonometry  Operator=cos
  Product{2..5} (4 alike) : Product
  Scope1 : Scope  NumInputPorts=2
  Sin : Trigonometry
  Sum : Sum  Inputs=|+-
  Sum1 : Sum  Inputs=|++
  Transport Delay2 : TransportDelay  DelayTime=0.25/60
  id : Outport
  iq : Outport  Port=2
  wires:
  phase/1 -> Sin/1, Cos/1
  Product4/1 -> Sum1/1
  Product3/1 -> Sum/1
  Product5/1 -> Sum1/2
  Sin/1 -> Product5/2, Product3/2
  Sum/1 -> id/1
  Sum1/1 -> iq/1
  Iac/1 -> Transport Delay2/1, Product3/1, Product4/1, Scope1/1  "Current originl"
  Transport Delay2/1 -> Scope1/2, Product5/1, Product2/1  "Current delay"
  Cos/1 -> Product2/2, Product4/2
  Product2/1 -> Sum/2

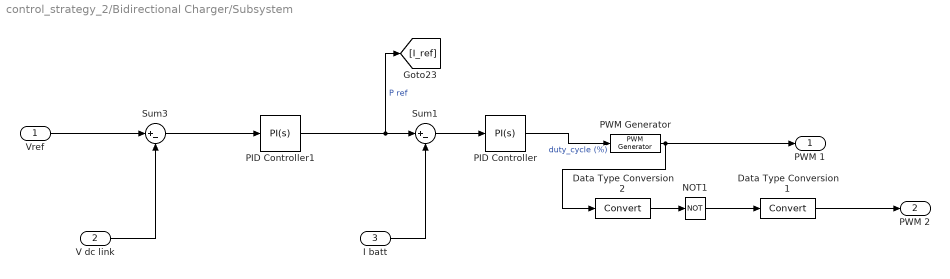
== system control_strategy_2/Bidirectional Charger/Subsystem ==
  Vref : Inport
  V dc link : Inport  Port=2
  I batt : Inport  Port=3
  Data Type Conversion1 : DataTypeConversion  SaturateOnIntegerOverflow=off  RndMeth=Floor
  Data Type Conversion2 : DataTypeConversion  SaturateOnIntegerOverflow=off  RndMeth=Floor
  NOT1 : Logic  Operator=NOT  IconShape=distinctive  AllPortsSameDT=off  OutDataTypeStr=boolean
  PID Controller : slpidlib/PID Controller  Controller=PI  Form=Parallel  TimeDomain=Continuous-time  UseExternalTs=off  SampleTime=-1  IntegratorMethod=Forward Euler  FilterMethod=Forward Euler  ControllerParametersSource=internal  P=KPi  I=KIi  UseKiTs=off  D=0  UseExternalDerivativeSource=off  N=100  UseFilter=on  TunerSelectOption=Transfer Function Based (PID Tuner App)  InitialConditionSource=internal  InitialConditionForIntegrator=0  InitialConditionForFilter=0  DifferentiatorICPrevScaledInput=0  ExternalReset=none  TrackingMode=off  Kt=1  LimitOutput=on  SatLimitsSource=internal  UpperSaturationLimit=1  LowerSaturationLimit=0  LinearizeAsGain=on  AntiWindupMode=none  Kb=1  LimitIntegrator=off  UpperIntegratorSaturationLimit=inf  LowerIntegratorSaturationLimit=-inf  POutMin=[]  POutMax=[]  IOutMin=[]  IOutMax=[]  DOutMin=[]  DOutMax=[]  NOutMin=[]  NOutMax=[]  SumOutMin=[]  SumOutMax=[]  SaturationOutMin=[]  SaturationOutMax=[]  PParamMin=[]  PParamMax=[]  IParamMin=[]  IParamMax=[]  DParamMin=[]  DParamMax=[]  NParamMin=[]  NParamMax=[]  KbParamMin=[]  KbParamMax=[]  KtParamMin=[]  KtParamMax=[]  KbOutMin=[]  KbOutMax=[]  KtOutMin=[]  KtOutMax=[]  IntegratorOutMin=[]  IntegratorOutMax=[]  FilterOutMin=[]  FilterOutMax=[]  SumI1OutMin=[]  SumI1OutMax=[]  SumI2OutMin=[]  SumI2OutMax=[]  SumI3OutMin=[]  SumI3OutMax=[]  SumI4OutMin=[]  SumI4OutMax=[]  SumDOutMin=[]  SumDOutMax=[]  DifferentiatorOutMin=[]  DifferentiatorOutMax=[]  FilterDiffOutCoefMin=[]  FilterDiffOutCoefMax=[]  ReciprocalOutMin=[]  ReciprocalOutMax=[]  SumDenOutMin=[]  SumDenOutMax=[]  SumNumOutMin=[]  SumNumOutMax=[]  DivideOutMin=[]  DivideOutMax=[]  UdiffTsProdOutMin=[]  UdiffTsProdOutMax=[]  NTsProdOutMin=[]  NTsProdOutMax=[]  UintegralTsProdOutMin=[]  UintegralTsProdOutMax=[]  UngainTsProdOutMin=[]  UngainTsProdOutMax=[]  ClampingZeroOutDataTypeStr=Inherit: Inherit via back propagation  ClampingZeroOutMin=[]  ClampingZeroOutMax=[]  FilterDenConstantOutDataTypeStr=Inherit: Inherit via back propagation  FilterDenConstantOutMin=[]  FilterDenConstantOutMax=[]  PCopyOutDataTypeStr=Inherit: Inherit via back propagation  PCopyOutMin=[]  PCopyOutMax=[]  NCopyOutDataTypeStr=Inherit: Inherit via back propagation  NCopyOutMin=[]  NCopyOutMax=[]  IntegratorContinuousStateAttributes=''  IntegratorStateMustResolveToSignalObject=off  IntegratorRTWStateStorageClass=Auto  FilterContinuousStateAttributes=''  FilterStateMustResolveToSignalObject=off  FilterRTWStateStorageClass=Auto  ParallelPVariant=InternalParameters  IdealPVariant=Disabled  IVariant=InternalParameters  DVariant=Disabled  IntegratorVariant=Continuous  SatVariant=Enabled  AWVariant=Passthrough  PCopyVariant=Disabled  TRVariant=Disabled  FdbkBlocksVariant=Forward  IdealPFdbkVariant=Disabled  SatFdbkVariant=Disabled  DerivativeFilterVariant=Disabled  NVariant=Disabled  NCopyVariant=Disabled_SignalSpec  FilterICVariant=Disabled  IntegratorICVariant=InternalICs  ExternalResetVariant=Disabled  TRSumVariant=Passthrough  SumFdbkVariant=Disabled  SumVariant=Sum_PI  TsampFilterVariant=InternalTs  TsampNgainVariant=Passthrough  TsampIntegralVariant=Disabled_SignalSpec  ExternalSaturationOutDataTypeStr=Inherit: Same as second input  DerivativeSourceVariant=Disabled  PreIntVariant=InternalPreInt
  PID Controller1 : slpidlib/PID Controller  Controller=PI  Form=Parallel  TimeDomain=Continuous-time  UseExternalTs=off  SampleTime=-1  IntegratorMethod=Forward Euler  FilterMethod=Forward Euler  ControllerParametersSource=internal  P=KP_out  I=KI_out  UseKiTs=off  D=0  UseExternalDerivativeSource=off  N=100  UseFilter=on  TunerSelectOption=Transfer Function Based (PID Tuner App)  InitialConditionSource=internal  InitialConditionForIntegrator=0  InitialConditionForFilter=0  DifferentiatorICPrevScaledInput=0  ExternalReset=none  TrackingMode=off  Kt=1  LimitOutput=on  SatLimitsSource=internal  UpperSaturationLimit=20  LowerSaturationLimit=-20  LinearizeAsGain=on  AntiWindupMode=none  Kb=1  LimitIntegrator=off  UpperIntegratorSaturationLimit=inf  LowerIntegratorSaturationLimit=-inf  POutMin=[]  POutMax=[]  IOutMin=[]  IOutMax=[]  DOutMin=[]  DOutMax=[]  NOutMin=[]  NOutMax=[]  SumOutMin=[]  SumOutMax=[]  SaturationOutMin=[]  SaturationOutMax=[]  PParamMin=[]  PParamMax=[]  IParamMin=[]  IParamMax=[]  DParamMin=[]  DParamMax=[]  NParamMin=[]  NParamMax=[]  KbParamMin=[]  KbParamMax=[]  KtParamMin=[]  KtParamMax=[]  KbOutMin=[]  KbOutMax=[]  KtOutMin=[]  KtOutMax=[]  IntegratorOutMin=[]  IntegratorOutMax=[]  FilterOutMin=[]  FilterOutMax=[]  SumI1OutMin=[]  SumI1OutMax=[]  SumI2OutMin=[]  SumI2OutMax=[]  SumI3OutMin=[]  SumI3OutMax=[]  SumI4OutMin=[]  SumI4OutMax=[]  SumDOutMin=[]  SumDOutMax=[]  DifferentiatorOutMin=[]  DifferentiatorOutMax=[]  FilterDiffOutCoefMin=[]  FilterDiffOutCoefMax=[]  ReciprocalOutMin=[]  ReciprocalOutMax=[]  SumDenOutMin=[]  SumDenOutMax=[]  SumNumOutMin=[]  SumNumOutMax=[]  DivideOutMin=[]  DivideOutMax=[]  UdiffTsProdOutMin=[]  UdiffTsProdOutMax=[]  NTsProdOutMin=[]  NTsProdOutMax=[]  UintegralTsProdOutMin=[]  UintegralTsProdOutMax=[]  UngainTsProdOutMin=[]  UngainTsProdOutMax=[]  ClampingZeroOutDataTypeStr=Inherit: Inherit via back propagation  ClampingZeroOutMin=[]  ClampingZeroOutMax=[]  FilterDenConstantOutDataTypeStr=Inherit: Inherit via back propagation  FilterDenConstantOutMin=[]  FilterDenConstantOutMax=[]  PCopyOutDataTypeStr=Inherit: Inherit via back propagation  PCopyOutMin=[]  PCopyOutMax=[]  NCopyOutDataTypeStr=Inherit: Inherit via back propagation  NCopyOutMin=[]  NCopyOutMax=[]  IntegratorContinuousStateAttributes=''  IntegratorStateMustResolveToSignalObject=off  IntegratorRTWStateStorageClass=Auto  FilterContinuousStateAttributes=''  FilterStateMustResolveToSignalObject=off  FilterRTWStateStorageClass=Auto  ParallelPVariant=InternalParameters  IdealPVariant=Disabled  IVariant=InternalParameters  DVariant=Disabled  IntegratorVariant=Continuous  SatVariant=Enabled  AWVariant=Passthrough  PCopyVariant=Disabled  TRVariant=Disabled  FdbkBlocksVariant=Forward  IdealPFdbkVariant=Disabled  SatFdbkVariant=Disabled  DerivativeFilterVariant=Disabled  NVariant=Disabled  NCopyVariant=Disabled_SignalSpec  FilterICVariant=Disabled  IntegratorICVariant=InternalICs  ExternalResetVariant=Disabled  TRSumVariant=Passthrough  SumFdbkVariant=Disabled  SumVariant=Sum_PI  TsampFilterVariant=InternalTs  TsampNgainVariant=Passthrough  TsampIntegralVariant=Disabled_SignalSpec  ExternalSaturationOutDataTypeStr=Inherit: Same as second input  DerivativeSourceVariant=Disabled  PreIntVariant=InternalPreInt
  PWM Generator : eePwmGenerator/PWM Generator  CarrCount=Up  Tper=Ts  Tdelay=0  Ts=0
  Sum1 : Sum  Inputs=|+-
  Sum3 : Sum  Inputs=|+-
  PWM 1 : Outport
  PWM 2 : Outport  Port=2
  wires:
  PID Controller/1 -> PWM Generator/1  "duty_cycle (%)"
  Vref/1 -> Sum3/1
  Sum3/1 -> PID Controller1/1
  NOT1/1 -> Data Type Conversion1/1
  PID Controller1/1 -> [I_ref], Sum1/1  "P ref"
  PWM Generator/1 -> PWM 1/1, Data Type Conversion2/1
  Sum1/1 -> PID Controller/1
  Data Type Conversion2/1 -> NOT1/1
  Data Type Conversion1/1 -> PWM 2/1
  V dc link/1 -> Sum3/2
  I batt/1 -> Sum1/2

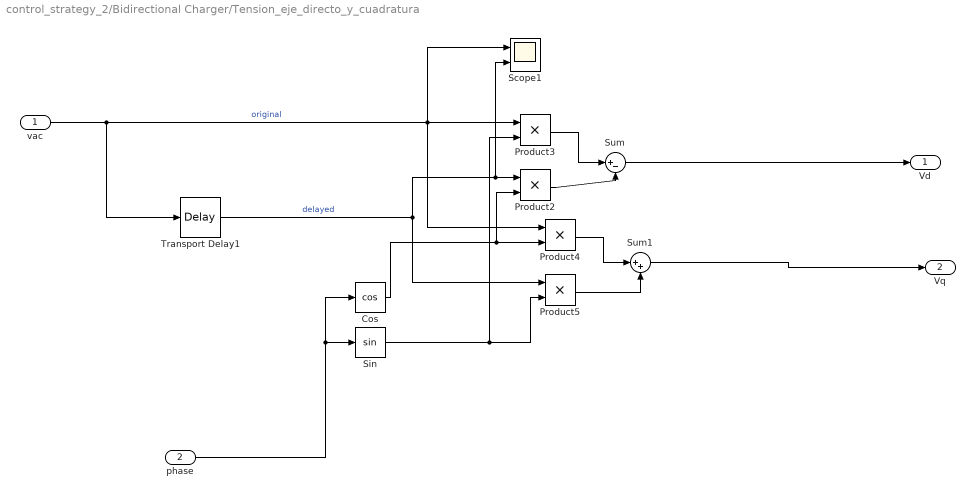
== system control_strategy_2/Bidirectional Charger/Tension_eje_directo_y_cuadratura ==
  vac : Inport
  phase : Inport  Port=2
  Cos : Trigonometry  Operator=cos
  Product{2..5} (4 alike) : Product
  Scope1 : Scope  NumInputPorts=2
  Sin : Trigonometry
  Sum : Sum  Inputs=|+-
  Sum1 : Sum  Inputs=|++
  Transport Delay1 : TransportDelay  DelayTime=0.25/60
  Vd : Outport
  Vq : Outport  Port=2
  wires:
  Product2/1 -> Sum/2
  Cos/1 -> Product4/2, Product2/2
  Transport Delay1/1 -> Scope1/2, Product2/1, Product5/1  "delayed"
  vac/1 -> Transport Delay1/1, Product4/1, Product3/1, Scope1/1  "original"
  Sum1/1 -> Vq/1
  Sum/1 -> Vd/1
  Sin/1 -> Product3/2, Product5/2
  Product5/1 -> Sum1/2
  Product3/1 -> Sum/1
  Product4/1 -> Sum1/1
  phase/1 -> Cos/1, Sin/1

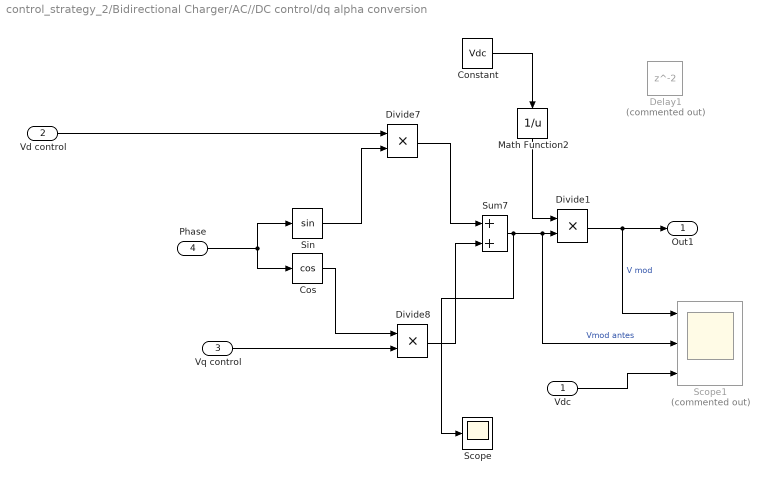
== system control_strategy_2/Bidirectional Charger/AC//DC control/dq alpha conversion ==
  Vdc : Inport
  Vd control : Inport  Port=2
  Vq control : Inport  Port=3
  Phase : Inport  Port=4
  Constant : Constant  Value=Vdc
  Cos : Trigonometry  Operator=cos
  Delay1 : Delay  Commented=on
  Divide1 : Product  Inputs=**
  Divide7 : Product  Inputs=**
  Divide8 : Product  Inputs=**
  Math Function2 : Math  Operator=reciprocal
  Scope : Scope
  Scope1 : Scope  Commented=on  NumInputPorts=3
  Sin : Trigonometry
  Sum7 : Sum
  Out1 : Outport
  wires:
  Cos/1 -> Divide8/1
  Sin/1 -> Divide7/2
  Vd control/1 -> Divide7/1
  Divide8/1 -> Sum7/2
  Divide7/1 -> Sum7/1
  Phase/1 -> Cos/1, Sin/1
  Vq control/1 -> Divide8/2
  Sum7/1 -> Scope/1, Scope1/2, Divide1/2  "Vmod antes"
  Divide1/1 -> Scope1/1, Out1/1  "V mod"
  Vdc/1 -> Scope1/3
  Math Function2/1 -> Divide1/1
  Constant/1 -> Math Function2/1
